simulink model "jacobian_test"  (R2018a)
settings: Solver=VariableStepAuto  StartTime=0.0  StopTime=10.0  RelTol=1e-3
settings Model: Creator=nalha  LastModifiedBy=nalha

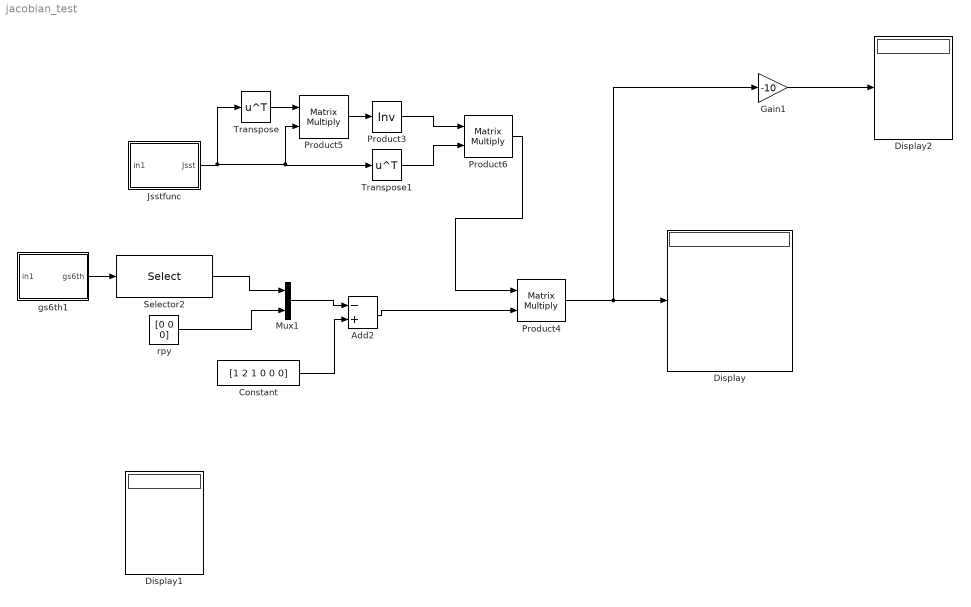
== system jacobian_test ==
  Add2 : Sum  Inputs=-+
  Constant : Constant  Value=[1 2 1 0 0 0]
  Display : Display
  Display1 : Display
  Display2 : Display
  Gain1 : Gain  Gain=-10
  Jsstfunc : MATLAB Function  TreatAsAtomicUnit=on
  Mux1 : Mux  Inputs=2
  Product3 : Product  Inputs=/  Multiplication=Matrix(*)
  Product4 : Product  Inputs=**  Multiplication=Matrix(*)
  Product5 : Product  Inputs=**  Multiplication=Matrix(*)
  Product6 : Product  Inputs=**  Multiplication=Matrix(*)
  Selector2 : Selector  NumberOfDimensions=2  InputPortWidth=3  IndexOptions=Index vector (dialog),Index vector (dialog)  Indices=[1 2 3],4  OutputSizes=1,1
  Transpose : Math  Operator=transpose  SaturateOnIntegerOverflow=on
  Transpose1 : Math  Operator=transpose  SaturateOnIntegerOverflow=on
  gs6th1 : MATLAB Function  TreatAsAtomicUnit=on
  "rpy " : Constant  Value=[0 0 0]
  wires:
  gs6th1/1(gs6th) -> Selector2/1
  Jsstfunc/1(Jsst) -> Transpose1/1, Product5/2, Transpose/1
  Selector2/1 -> Mux1/1
  Product6/1 -> Product4/1
  Product5/1 -> Product3/1
  Gain1/1 -> Display2/1
  "rpy "/1 -> Mux1/2
  Product4/1 -> Gain1/1, Display/1
  Add2/1 -> Product4/2
  Mux1/1 -> Add2/1
  Constant/1 -> Add2/2
  Transpose/1 -> Product5/1
  Transpose1/1 -> Product6/2
  Product3/1 -> Product6/1

== matlab function jacobian_test/Jsstfunc ==
  data: in1 input; Jsst output
function Jsst = Jsstfunc(in1)
%#codegen

%    This function was generated by the Symbolic Math Toolbox version 8.1.
%    10-May-2018 02:30:39

th1 = in1(1,:);
th2 = in1(2,:);
th3 = in1(3,:);
th4 = in1(4,:);
th5 = in1(5,:);
t2 = sin(th4);
t3 = th3+3.0./1.0e1;
t4 = cos(th4);
t5 = th3.*1.0e1;
t6 = sin(th5);
t7 = t5-t6.*5.0+3.0;
t8 = t2.*(1.0./2.0e1);
t9 = t4.*th2;
Jsst = reshape([1.0,0.0,0.0,0.0,0.0,0.0,0.0,1.0,0.0,0.0,0.0,0.0,0.0,0.0,1.0,0.0,0.0,0.0,th2,-th1+1.0./2.0e1,0.0,0.0,0.0,1.0,t2.*t3,-t3.*t4,t8+t9-t2.*th1,-t4,-t2,0.0,t2.*t7.*(1.0./1.0e1),t4.*t7.*(-1.0./1.0e1),t8+t9+cos(th5).*(1.0./2.0)-t2.*th1,-t4,-t2,0.0],[6,6]);

== matlab function jacobian_test/gs6th1 ==
  data: in1 input; gs6th output
function gs6th = gs6th(in1)
%#codegen

%    This function was generated by the Symbolic Math Toolbox version 8.1.
%    10-May-2018 02:30:37

th1 = in1(1,:);
th2 = in1(2,:);
th3 = in1(3,:);
th4 = in1(4,:);
th5 = in1(5,:);
th6 = in1(6,:);
t2 = th5+th6;
t3 = sin(th4);
t4 = cos(th4);
t5 = cos(th5);
t6 = cos(t2);
t7 = sin(t2);
t8 = sin(th5);
t9 = sin(th6);
t10 = cos(th6);
gs6th = reshape([t4,t3,0.0,0.0,-t3.*t6,t4.*t6,-t7,0.0,-t3.*t7,t4.*t7,t6,0.0,t4.*(1.0./1.0e1)+th1-t3.*t5.*(1.0./2.0)-t3.*t5.*t10.*(1.0./4.0)+t3.*t8.*t9.*(1.0./4.0)-1.0./2.0e1,t3.*(1.0./1.0e1)+th2+t4.*t5.*(1.0./2.0)+t4.*t5.*t10.*(1.0./4.0)-t4.*t8.*t9.*(1.0./4.0),t7.*(-1.0./4.0)-t8.*(1.0./2.0)+th3+3.0./1.0e1,1.0],[4,4]);
